simulink library "xpckeithleylib"  (Simulink 6.0)
settings: Solver=ode45  SolverMode=SingleTasking  StartTime=0.0  StopTime=10.0  RelTol=1e-3
values from neighbouring files (symbols this model uses):
  channels = round(channels)    [mbwaudpmc.m]
undefined symbols (not defined in the file or in its folder): madkpci1800, mdakpci1800, mdiokpci1800
settings Model: Creator=adowd  LastModifiedBy=gweast
settings DataIOCC: SignalLoggingName=logsOut
settings OptimizationCC: BooleanDataType=off
settings DebuggingCC: CheckExecutionContextPreStartOutputMsg=on  CheckExecutionContextRuntimeOutputMsg=on  SolverPrmCheckMsg=none
settings HardwareCC: TargetUnknown=on
settings GRTTargetCC: UtilityFuncGeneration=Automatic  LifeSpan=inf
settings SFSimCC: SFSimApplyToAllLibs=on  SFSimBuildMode=Incremental

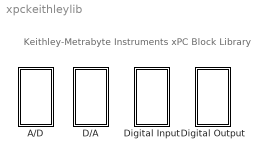
== system xpckeithleylib ==
  note: Keithley-Metrabyte Instruments xPC Block Library
  A/D : Subsystem  EnableExecutionContextPropagation=on
  D/A : Subsystem  EnableExecutionContextPropagation=on
  Digital Input : Subsystem  EnableExecutionContextPropagation=on
  Digital Output : Subsystem  EnableExecutionContextPropagation=on

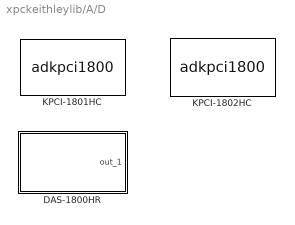
== system xpckeithleylib/A/D ==
  "DAS-1800HR " : Subsystem  EnableExecutionContextPropagation=on  mask(Analog Input Module){channels=[1], gain=[1], range=Bipolar, mux=Differential (8 channels), sampletime=0.001, baseaddress=0x300}
      mask prompts: channels "Channel vector:"; gain "Gain vector (1,2,4,8):"; range "Range vector:"; mux "Input coupling:"; sampletime "Sample time:"; baseaddress "Base address (i.e. 0xd000):"
      mask help:
      | Keithley Metrabyte
      | DAS-1800HR
      | Analog Input
      mask init:
      | baseaddress=hex2dec(baseaddress(3:end));
      mask Help: helpview(fullfile(docroot, 'mapfiles', 'xpc.map'), 'KeithleyMetrabyte_DAS-1800HR_AD')
      mask StyleString: edit,edit,popup(Bipolar|Unipolar),popup(Differential (8 channels)|Single-ended (16 channels)|Single-ended common mode (16 channels)),edit,edit
      mask Display: disp('DAS-1800HR\nKeithley Metrabyte\nAnalog Input')
  "KPCI-1801HC " : S-Function  InitFcn=madkpci1800(1);  FunctionName=adkpci1800  Parameters="channel, range, coupling, sampletime, slot,  boardType"  mask(adkpci1801hc){channel=[1], range=[-5], coupling=[0], sampletime=0.001, slot=-1}
      mask prompts: channel "Channel vector:"; range "Range vector:"; coupling "Input coupling vector (0: Single-ended, 1: Differential):"; sampletime "Sample time:"; slot "PCI slot (-1: autosearch):"
      mask help:
      | KPCI-1801HC
      | Keithley
      | Analog Input
      mask init:
      | boardType=2;
      | madkpci1800(2, channel, range, coupling, slot, boardType);
      mask Help: helpview(fullfile(docroot, 'mapfiles', 'xpc.map'), 'KeithleyMetrabyte_KPCI-1801HC_AD')
      mask Display: disp('KPCI-1801HC\nKeithley\nAnalog Input');port_label('output',1,'1');
  "KPCI-1802HC " : S-Function  InitFcn=madkpci1800(1);  FunctionName=adkpci1800  Parameters="channel, range, coupling, sampletime, slot,  boardType"  mask(adkpci1802hc){channel=[1], range=[-10], coupling=[0], sampletime=0.001, slot=-1}
      mask prompts: channel "Channel vector:"; range "Range vector:"; coupling "Input coupling vector (0: Single-ended, 1: Differential):"; sampletime "Sample time:"; slot "PCI slot (-1: autosearch):"
      mask help:
      | KPCI-1802HC
      | Keithley
      | Analog Input
      mask init:
      | boardType=1;
      | madkpci1800(2, channel, range, coupling, slot, boardType);
      mask Help: helpview(fullfile(docroot, 'mapfiles', 'xpc.map'), 'KeithleyMetrabyte_KPCI-1802HC_AD')
      mask Display: disp('KPCI-1802HC\nKeithley\nAnalog Input');port_label('output',1,'1');

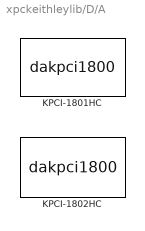
== system xpckeithleylib/D/A ==
  "KPCI-1801HC " : S-Function  InitFcn=mdakpci1800(1);  FunctionName=dakpci1800  Parameters="channel, reset, initValue, sampletime, slot,  boardType"  mask(dakpci1801hc){channel=[1], reset=[1], initValue=[0], sampletime=0.001, slot=-1}
      mask prompts: channel "Channel vector:"; reset "Reset vector:"; initValue "Initial value vector:"; sampletime "Sample time:"; slot "PCI slot (-1: autosearch):"
      mask help:
      | KPCI-1801HC
      | Keithley
      | Analog Output
      mask init:
      | boardType=2;
      | range=-10; coupling=0;
      | [reset, initValue, range, coupling] = mdakpci1800(2, channel, reset, initValue, range, coupling, slot, boardType);
      mask Help: helpview(fullfile(docroot, 'mapfiles', 'xpc.map'), 'KeithleyMetrabyte_KPCI-1801HC_DA')
      mask Display: disp('KPCI-1801HC\nKeithley\nAnalog Output');port_label('input',1,'1');
  "KPCI-1802HC " : S-Function  InitFcn=mdakpci1800(1);  FunctionName=dakpci1800  Parameters="channel, reset, initValue, sampletime, slot,  boardType"  mask(dakpci1802hc){channel=[1], reset=[1], initValue=[0], sampletime=0.001, slot=-1}
      mask prompts: channel "Channel vector:"; reset "Reset vector:"; initValue "Initial value vector:"; sampletime "Sample time:"; slot "PCI slot (-1: autosearch):"
      mask help:
      | KPCI-1802HC
      | Keithley
      | Analog Output
      mask init:
      | boardType=1;
      | range=-10; coupling=0;
      | [reset, initValue, range, coupling] = mdakpci1800(2, channel, reset, initValue, range, coupling, slot, boardType);
      mask Help: helpview(fullfile(docroot, 'mapfiles', 'xpc.map'), 'KeithleyMetrabyte_KPCI-1802HC_DA')
      mask Display: disp('KPCI-1802HC\nKeithley\nAnalog Output');port_label('input',1,'1');

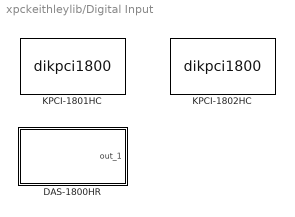
== system xpckeithleylib/Digital Input ==
  "DAS-1800HR " : Subsystem  EnableExecutionContextPropagation=on  mask(Digital Input Module){n_channels=1, sample_time=0.001, baseaddress=0x300}
      mask prompts: n_channels "Number of channels:"; sample_time "Sample time:"; baseaddress "Base address (i.e. 0xd000):"
      mask help:
      | Keithley Metrabyte
      | DAS-1800HR
      | Digital Input
      mask init:
      | baseaddress=hex2dec(baseaddress(3:end));
      mask Help: helpview(fullfile(docroot, 'mapfiles', 'xpc.map'), 'KeithleyMetrabyte_DAS-1800HR_DIN')
      mask Display: disp('DAS-1800HR\nKeithley Metrabyte\nDigital Input')
  "KPCI-1801HC " : S-Function  InitFcn=mdiokpci1800(1);  FunctionName=dikpci1800  Parameters=channel,sampletime,slot, control, boardType  mask(dikpci1801hc){channel=[1], sampletime=0.001, slot=-1}
      mask prompts: channel "Channel vector:"; sampletime "Sample time:"; slot "PCI slot (-1: autosearch):"
      mask help:
      | KPCI-1801HC
      | Keithley
      | Digital Input
      mask init:
      | control=0;
      | boardType=2;
      | mdiokpci1800(2, channel,slot,1,boardType);
      mask Help: helpview(fullfile(docroot, 'mapfiles', 'xpc.map'), 'KeithleyMetrabyte_KPCI-1801HC_DIN')
      mask Display: disp('KPCI-1801HC\nKeithley\nDigital Input');port_label('output',1,'1');
  "KPCI-1802HC " : S-Function  InitFcn=mdiokpci1800(1);  FunctionName=dikpci1800  Parameters=channel,sampletime,slot, control, boardType  mask(dikpci1802hc){channel=[1], sampletime=0.001, slot=-1}
      mask prompts: channel "Channel vector:"; sampletime "Sample time:"; slot "PCI slot (-1: autosearch):"
      mask help:
      | KPCI-1802HC
      | Keithley
      | Digital Input
      mask init:
      | control=0;
      | boardType=1;
      | mdiokpci1800(2, channel,slot,1,boardType);
      mask Help: helpview(fullfile(docroot, 'mapfiles', 'xpc.map'), 'KeithleyMetrabyte_KPCI-1802HC_DIN')
      mask Display: disp('KPCI-1802HC\nKeithley\nDigital Input');port_label('output',1,'1');

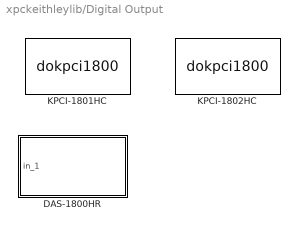
== system xpckeithleylib/Digital Output ==
  "DAS-1800HR " : Subsystem  EnableExecutionContextPropagation=on  mask(Digital Output Module){n_channels=1, sample_time=0.001, baseaddress=0x300}
      mask prompts: n_channels "Number of channels:"; sample_time "Sample time:"; baseaddress "Base address (i.e. 0xd000):"
      mask help:
      | Keithley Metrabyte
      | DAS-1800HR
      | Digital Output
      mask init:
      | baseaddress=hex2dec(baseaddress(3:end));
      mask Help: helpview(fullfile(docroot, 'mapfiles', 'xpc.map'), 'KeithleyMetrabyte_DAS-1800HR_DOUT')
      mask Display: disp('DAS-1800HR\nKeithley Metrabyte\nDigital Output')
  "KPCI-1801HC " : S-Function  InitFcn=mdiokpci1800(1);  FunctionName=dokpci1800  Parameters=channel, reset, initValue, sampletime, slot, control, boardType  mask(dokpci1801hc){channel=[1], reset=[1], initValue=[0], sampletime=0.001, slot=-1}
      mask prompts: channel "Channel vector:"; reset "Reset vector:"; initValue "Initial value vector:"; sampletime "Sample time:"; slot "PCI slot (-1: autosearch):"
      mask help:
      | KPCI-1801HC
      | Keithley
      | Digital Output
      mask init:
      | control=0;
      | boardType=2;
      | [reset, initValue] = mdiokpci1800(2, channel, slot, 2, boardType, reset, initValue);
      mask Help: helpview(fullfile(docroot, 'mapfiles', 'xpc.map'), 'KeithleyMetrabyte_KPCI-1801HC_DOUT')
      mask Display: disp('KPCI-1801HC\nKeithley\nDigital Output');port_label('input',1,'1');
  "KPCI-1802HC " : S-Function  InitFcn=mdiokpci1800(1);  FunctionName=dokpci1800  Parameters=channel, reset, initValue, sampletime, slot, control, boardType  mask(dokpci1802hc){channel=[1], reset=[1], initValue=[0], sampletime=0.001, slot=-1}
      mask prompts: channel "Channel vector:"; reset "Reset vector:"; initValue "Initial value vector:"; sampletime "Sample time:"; slot "PCI slot (-1: autosearch):"
      mask help:
      | KPCI-1802HC
      | Keithley
      | Digital Output
      mask init:
      | control=0;
      | boardType=1;
      | [reset, initValue] = mdiokpci1800(2, channel, slot, 2, boardType, reset, initValue);
      mask Help: helpview(fullfile(docroot, 'mapfiles', 'xpc.map'), 'KeithleyMetrabyte_KPCI-1802HC_DOUT')
      mask Display: disp('KPCI-1802HC\nKeithley\nDigital Output');port_label('input',1,'1');

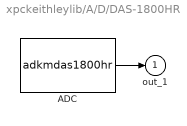
== system xpckeithleylib/A/D/DAS-1800HR  ==
  ADC : S-Function  FunctionName=adkmdas1800hr  Parameters=channels, gain, range, mux, sampletime, baseaddress
  out_1 : Outport  InitialOutput=0
  wires:
  ADC/1 -> out_1/1

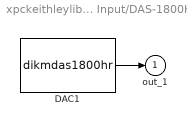
== system xpckeithleylib/Digital Input/DAS-1800HR  ==
  DAC1 : S-Function  FunctionName=dikmdas1800hr  Parameters=n_channels,sample_time,baseaddress
  out_1 : Outport  InitialOutput=0
  wires:
  DAC1/1 -> out_1/1

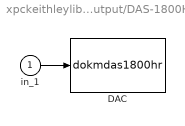
== system xpckeithleylib/Digital Output/DAS-1800HR  ==
  in_1 : Inport  LatchInput=off
  DAC : S-Function  FunctionName=dokmdas1800hr  Parameters=n_channels,sample_time,baseaddress
  wires:
  in_1/1 -> DAC/1
